simulink model "ADI"  (R2019b)
settings: Solver=FixedStepAuto  StartTime=0.0  StopTime=10.0  FixedStep=fixedStepSize  RelTol=1e-3
undefined symbols (not defined in the file): ADI_evChangesDuration, ADI_notAlways1Horizon, ADI_outputTorqueBound, ADI_subsystem1_downThreshold1, ADI_subsystem1_downThreshold2, ADI_subsystem1_downThreshold3, ADI_subsystem1_downThreshold4, ADI_subsystem1_evChangesDuration, ADI_subsystem1_gearOption1, ADI_subsystem1_gearOption2, ADI_subsystem1_speedThreshold, ADI_subsystem2_evChangesDuration, ADI_subsystem2_gear1, ADI_subsystem2_gear2, ADI_subsystem2_notAlwaysHorizon, ADI_subsystem2_speedMin, ADI_subsystem3_downThreshold, ADI_subsystem3_gear, ADI_subsystem3_gearSelectionState, ADI_subsystem3_impellerTorque, ADI_subsystem3_RPM, ADI_subsystem3_upThreshold, ADI_subsystem4_downThreshold, ADI_subsystem4_gear, ADI_subsystem4_gearSelectionState, ADI_subsystem4_notAlways1Horizon, ADI_subsystem4_notAlwaysHorizon, ADI_subsystem4_RPM, ADI_subsystem4_throttle, ADI_subsystem4_upThreshold, ADI_subsystem5_evChanges1Duration, ADI_subsystem5_evChangesDuration, ADI_subsystem5_notAlwaysHorizon, ADI_subsystem5_speedThreshold, fixedStepSize
libraries: simulink x11
settings Model: Creator=JEDDELAN  LastModifiedBy=alex
settings DataIOCC: ReturnWorkspaceOutputs=off
settings DebuggingCC: ArithmeticOperatorsInVariantConditions=warning
settings SFSimCC: SimUseLocalCustomCode=off  CustomCodeUndefinedFunction=UseInterfaceOnly
settings RTWCC: RTWUseLocalCustomCode=off

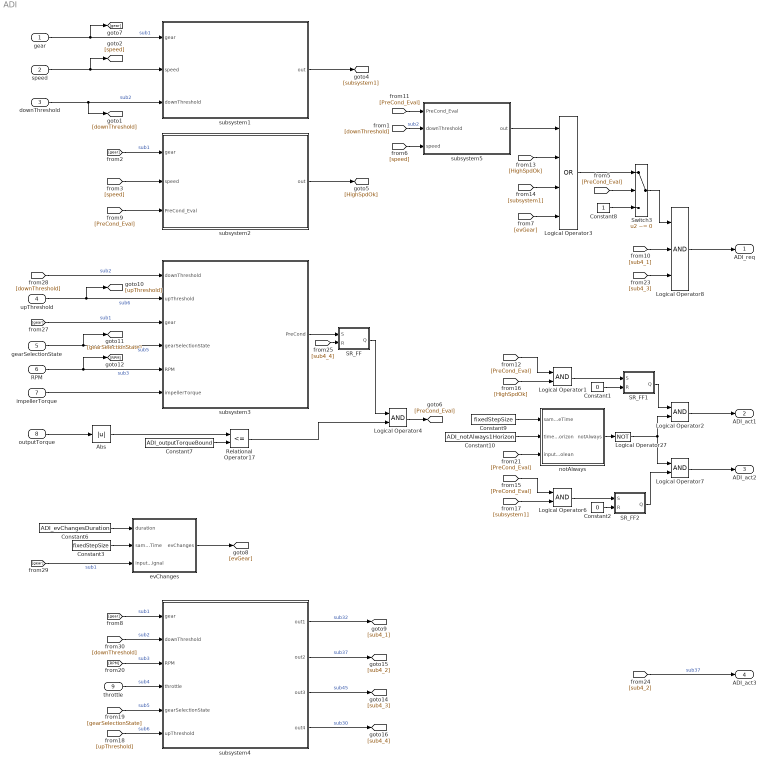
== system ADI ==
  gear : Inport
  speed : Inport  Port=2
  downThreshold : Inport  Port=3
  upThreshold : Inport  Port=4
  gearSelectionState : Inport  Port=5
  RPM : Inport  Port=6
  impellerTorque : Inport  Port=7
  outputTorque : Inport  Port=8
  throttle : Inport  Port=9
  Abs : Abs
  Constant1 : Constant  Value=0  OutDataTypeStr=boolean
  Constant10 : Constant  Value=ADI_notAlways1Horizon
  Constant2 : Constant  Value=0  OutDataTypeStr=boolean
  Constant3 : Constant  Value=fixedStepSize
  Constant6 : Constant  Value=ADI_evChangesDuration
  Constant7 : Constant  Value=ADI_outputTorqueBound
  Constant8 : Constant
  Constant9 : Constant  Value=fixedStepSize
  Logical Operator{1..2,4,6..7} (5 alike) : Logic  AllPortsSameDT=off  OutDataTypeStr=boolean
  Logical Operator27 : Logic  Operator=NOT  AllPortsSameDT=off  OutDataTypeStr=boolean
  Logical Operator3 : Logic  Operator=OR  Inputs=4  AllPortsSameDT=off  OutDataTypeStr=boolean
  Logical Operator8 : Logic  Inputs=3  AllPortsSameDT=off  OutDataTypeStr=boolean
  Relational Operator17 : RelationalOperator  Operator=<=  OutDataTypeStr=boolean  RndMeth=Nearest
  SR_FF : Subsystem
      settings: CopyFcn=set_param(gcbh,'LinkStatus','none');
  SR_FF1 : Subsystem
      settings: CopyFcn=set_param(gcbh,'LinkStatus','none');
  SR_FF2 : Subsystem
      settings: CopyFcn=set_param(gcbh,'LinkStatus','none');
  Switch3 : Switch  Criteria=u2 ~= 0
  evChanges : Subsystem
      settings: CopyFcn=set_param(gcbh,'LinkStatus','none');
  notAlways : Subsystem
      settings: CopyFcn=set_param(gcbh,'LinkStatus','none');
  subsystem1 : Subsystem
  subsystem2 : Subsystem
  subsystem3 : Subsystem
  subsystem4 : Subsystem
  subsystem5 : Subsystem
  ADI_req : Outport  OutDataTypeStr=boolean  PortDimensions=1  VectorParamsAs1DForOutWhenUnconnected=off
  ADI_act1 : Outport  Port=2  OutDataTypeStr=boolean  PortDimensions=1  VectorParamsAs1DForOutWhenUnconnected=off
  ADI_act2 : Outport  Port=3  OutDataTypeStr=boolean  PortDimensions=1  VectorParamsAs1DForOutWhenUnconnected=off
  ADI_act3 : Outport  Port=4  OutDataTypeStr=boolean  PortDimensions=1  VectorParamsAs1DForOutWhenUnconnected=off
  wires:
  evChanges/1(evChanges) -> [evGear]
  [gear] -> evChanges/3(inputSignal)  "sub1"
  Relational Operator17/1 -> Logical Operator4/2
  subsystem4/2(out2) -> [sub4_2]  "sub37"
  Constant10/1 -> notAlways/2(timeHorizon)
  [downThreshold] -> subsystem3/1(downThreshold)  "sub2"
  SR_FF/1(Q) -> Logical Operator4/1
  subsystem4/4(out4) -> [sub4_4]  "sub30"
  [subsystem1] -> Logical Operator6/2
  subsystem3/1(PreCond) -> SR_FF/1(S)
  [sub4_4] -> SR_FF/2(R)
  [downThreshold] -> subsystem5/2(downThreshold)  "sub2"
  [HighSpdOk] -> Logical Operator1/2
  [upThreshold] -> subsystem4/6(upThreshold)  "sub6"
  Logical Operator3/1 -> Switch3/1
  subsystem4/3(out3) -> [sub4_3]  "sub45"
  impellerTorque/1 -> subsystem3/6(impellerTorque)
  [sub4_3] -> Logical Operator8/3
  [PreCond_Eval] -> subsystem2/3(PreCond_Eval)
  [sub4_1] -> Logical Operator8/2
  [gear] -> subsystem4/1(gear)  "sub1"
  Abs/1 -> Relational Operator17/1
  [downThreshold] -> subsystem4/2(downThreshold)  "sub2"
  Constant6/1 -> evChanges/1(duration)
  [gear] -> subsystem2/1(gear)  "sub1"
  Logical Operator27/1 -> Logical Operator2/2, Logical Operator7/1
  speed/1 -> subsystem1/2("speed "), [speed]
  [speed] -> subsystem2/2(speed)
  gear/1 -> subsystem1/1(gear), [gear]  "sub1"
  [gear] -> subsystem3/3(gear)  "sub1"
  [sub4_2] -> ADI_act3/1  "sub37"
  [RPM] -> subsystem4/3(RPM)  "sub3"
  notAlways/1(notAlways) -> Logical Operator27/1
  [speed] -> subsystem5/3(speed)
  gearSelectionState/1 -> [gearSelectionState], subsystem3/4(gearSelectionState)  "sub5"
  Logical Operator8/1 -> ADI_req/1
  Logical Operator7/1 -> ADI_act2/1
  Logical Operator6/1 -> SR_FF2/1(S)
  RPM/1 -> [RPM], subsystem3/5(RPM)  "sub3"
  Constant7/1 -> Relational Operator17/2
  upThreshold/1 -> subsystem3/2(upThreshold), [upThreshold]  "sub6"
  downThreshold/1 -> subsystem1/3(downThreshold), [downThreshold]  "sub2"
  [PreCond_Eval] -> Switch3/2
  [gearSelectionState] -> subsystem4/5(gearSelectionState)  "sub5"
  throttle/1 -> subsystem4/4(throttle)  "sub4"
  Constant2/1 -> SR_FF2/2(R)
  [PreCond_Eval] -> Logical Operator1/1
  subsystem2/1(out) -> [HighSpdOk]
  Constant9/1 -> notAlways/1(sampleTime)
  Logical Operator4/1 -> [PreCond_Eval]
  subsystem1/1(out) -> [subsystem1]
  [PreCond_Eval] -> Logical Operator6/1
  [evGear] -> Logical Operator3/4
  SR_FF2/1(Q) -> Logical Operator7/2
  SR_FF1/1(Q) -> Logical Operator2/1
  Constant8/1 -> Switch3/3
  [HighSpdOk] -> Logical Operator3/2
  Logical Operator2/1 -> ADI_act1/1
  [subsystem1] -> Logical Operator3/3
  Switch3/1 -> Logical Operator8/1
  [PreCond_Eval] -> subsystem5/1(PreCond_Eval)
  subsystem4/1(out1) -> [sub4_1]  "sub32"
  Logical Operator1/1 -> SR_FF1/1(S)
  subsystem5/1(out) -> Logical Operator3/1
  [PreCond_Eval] -> notAlways/3(inputBoolean)
  outputTorque/1 -> Abs/1
  Constant3/1 -> evChanges/2(sampleTime)
  Constant1/1 -> SR_FF1/2(R)

== system ADI/SR_FF ==
  S : Inport  OutDataTypeStr=boolean
  R : Inport  Port=2  OutDataTypeStr=boolean
  LogOp1 : Logic  Tag=struct('inputs','1','comment',struct('text','','placement',1),'logdata',struct('maxnumvals',4096,'plotchannels',[],'loggingmode',3,'channels',1),'operator','NOT','output',struct('class','default','description','','address','','unit','-','name','$S_$B','variable','','type','Bool'),'date',733638.68643228011,'scalingvalid',0)  Operator=NOT  Inputs=1  OutDataTypeStr=boolean
  LogOp2 : Logic  Tag=struct('inputs','2','comment',struct('text','','placement',1),'logdata',struct('maxnumvals',4096,'plotchannels',[],'loggingmode',3,'channels',1),'operator','AND','output',struct('class','default','description','','address','','unit','-','name','$S_$B','variable','','type','Bool'),'date',733638.68643680552,'scalingvalid',0)  Operator=OR  OutDataTypeStr=boolean
  LogOp3 : Logic  Tag=struct('inputs','2','comment',struct('text','','placement',1),'logdata',struct('maxnumvals',4096,'plotchannels',[],'loggingmode',3,'channels',1),'operator','OR','output',struct('class','default','description','','address','','unit','-','name','$S_$B','variable','','type','Bool'),'date',733638.68644151615,'scalingvalid',0)  OutDataTypeStr=boolean
  UnitDelay1 : UnitDelay  Tag=struct('comment',struct('text','','placement',1),'logdata',struct('maxnumvals',4096,'plotchannels',[],'loggingmode',3,'channels',1),'output',struct('width',1,'name','$S_$B','unit','','type','Bool','offset',0,'max',NaN,'min',NaN,'freeze',1,'lsb',1,'arb',0,'class','default','address','','description','','autoscalingmode',1,'lowerheadroom',1,'upperheadroom',1,'headroomunit','bit','checkmin',0,'checkmax',0,'show',0,'variable','','scaling','','keepdatatype',1,'castoutput',0),'state',struct('variable','','description','','name','X_$S_$B','width',1,'address','','max',NaN,'min',NaN,'class','default','type','Bool','scaling','','lsb',1,'offset',0,'arb',0,'freeze',1,'unit','','initial','0'),'dt','-1','date',733638.68644640048,'scalingvalid',0)  SampleTime=-1  HasFrameUpgradeWarning=on
  Q : Outport  OutDataTypeStr=boolean  VectorParamsAs1DForOutWhenUnconnected=off
  wires:
  UnitDelay1/1 -> LogOp2/1  "UnitDelay1_3"
  S/1 -> LogOp2/2
  R/1 -> LogOp1/1
  LogOp2/1 -> LogOp3/1
  LogOp1/1 -> LogOp3/2
  LogOp3/1 -> UnitDelay1/1, Q/1

== system ADI/SR_FF1 ==
  S : Inport  OutDataTypeStr=boolean
  R : Inport  Port=2  OutDataTypeStr=boolean
  LogOp1 : Logic  Tag=struct('inputs','1','comment',struct('text','','placement',1),'logdata',struct('maxnumvals',4096,'plotchannels',[],'loggingmode',3,'channels',1),'operator','NOT','output',struct('class','default','description','','address','','unit','-','name','$S_$B','variable','','type','Bool'),'date',733638.68643228011,'scalingvalid',0)  Operator=NOT  Inputs=1  OutDataTypeStr=boolean
  LogOp2 : Logic  Tag=struct('inputs','2','comment',struct('text','','placement',1),'logdata',struct('maxnumvals',4096,'plotchannels',[],'loggingmode',3,'channels',1),'operator','AND','output',struct('class','default','description','','address','','unit','-','name','$S_$B','variable','','type','Bool'),'date',733638.68643680552,'scalingvalid',0)  Operator=OR  OutDataTypeStr=boolean
  LogOp3 : Logic  Tag=struct('inputs','2','comment',struct('text','','placement',1),'logdata',struct('maxnumvals',4096,'plotchannels',[],'loggingmode',3,'channels',1),'operator','OR','output',struct('class','default','description','','address','','unit','-','name','$S_$B','variable','','type','Bool'),'date',733638.68644151615,'scalingvalid',0)  OutDataTypeStr=boolean
  UnitDelay1 : UnitDelay  Tag=struct('comment',struct('text','','placement',1),'logdata',struct('maxnumvals',4096,'plotchannels',[],'loggingmode',3,'channels',1),'output',struct('width',1,'name','$S_$B','unit','','type','Bool','offset',0,'max',NaN,'min',NaN,'freeze',1,'lsb',1,'arb',0,'class','default','address','','description','','autoscalingmode',1,'lowerheadroom',1,'upperheadroom',1,'headroomunit','bit','checkmin',0,'checkmax',0,'show',0,'variable','','scaling','','keepdatatype',1,'castoutput',0),'state',struct('variable','','description','','name','X_$S_$B','width',1,'address','','max',NaN,'min',NaN,'class','default','type','Bool','scaling','','lsb',1,'offset',0,'arb',0,'freeze',1,'unit','','initial','0'),'dt','-1','date',733638.68644640048,'scalingvalid',0)  SampleTime=-1  HasFrameUpgradeWarning=on
  Q : Outport  OutDataTypeStr=boolean  VectorParamsAs1DForOutWhenUnconnected=off
  wires:
  UnitDelay1/1 -> LogOp2/1
  S/1 -> LogOp2/2
  R/1 -> LogOp1/1
  LogOp2/1 -> LogOp3/1
  LogOp1/1 -> LogOp3/2
  LogOp3/1 -> UnitDelay1/1, Q/1

== system ADI/SR_FF2 ==
  S : Inport  OutDataTypeStr=boolean
  R : Inport  Port=2  OutDataTypeStr=boolean
  LogOp1 : Logic  Tag=struct('inputs','1','comment',struct('text','','placement',1),'logdata',struct('maxnumvals',4096,'plotchannels',[],'loggingmode',3,'channels',1),'operator','NOT','output',struct('class','default','description','','address','','unit','-','name','$S_$B','variable','','type','Bool'),'date',733638.68643228011,'scalingvalid',0)  Operator=NOT  Inputs=1  OutDataTypeStr=boolean
  LogOp2 : Logic  Tag=struct('inputs','2','comment',struct('text','','placement',1),'logdata',struct('maxnumvals',4096,'plotchannels',[],'loggingmode',3,'channels',1),'operator','AND','output',struct('class','default','description','','address','','unit','-','name','$S_$B','variable','','type','Bool'),'date',733638.68643680552,'scalingvalid',0)  Operator=OR  OutDataTypeStr=boolean
  LogOp3 : Logic  Tag=struct('inputs','2','comment',struct('text','','placement',1),'logdata',struct('maxnumvals',4096,'plotchannels',[],'loggingmode',3,'channels',1),'operator','OR','output',struct('class','default','description','','address','','unit','-','name','$S_$B','variable','','type','Bool'),'date',733638.68644151615,'scalingvalid',0)  OutDataTypeStr=boolean
  UnitDelay1 : UnitDelay  Tag=struct('comment',struct('text','','placement',1),'logdata',struct('maxnumvals',4096,'plotchannels',[],'loggingmode',3,'channels',1),'output',struct('width',1,'name','$S_$B','unit','','type','Bool','offset',0,'max',NaN,'min',NaN,'freeze',1,'lsb',1,'arb',0,'class','default','address','','description','','autoscalingmode',1,'lowerheadroom',1,'upperheadroom',1,'headroomunit','bit','checkmin',0,'checkmax',0,'show',0,'variable','','scaling','','keepdatatype',1,'castoutput',0),'state',struct('variable','','description','','name','X_$S_$B','width',1,'address','','max',NaN,'min',NaN,'class','default','type','Bool','scaling','','lsb',1,'offset',0,'arb',0,'freeze',1,'unit','','initial','0'),'dt','-1','date',733638.68644640048,'scalingvalid',0)  SampleTime=-1  HasFrameUpgradeWarning=on
  Q : Outport  OutDataTypeStr=boolean  VectorParamsAs1DForOutWhenUnconnected=off
  wires:
  UnitDelay1/1 -> LogOp2/1
  S/1 -> LogOp2/2
  R/1 -> LogOp1/1
  LogOp2/1 -> LogOp3/1
  LogOp1/1 -> LogOp3/2
  LogOp3/1 -> UnitDelay1/1, Q/1

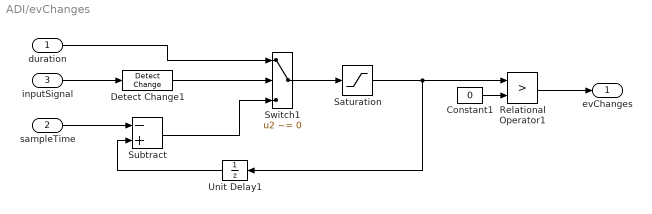
== system ADI/evChanges ==
  duration : Inport
  sampleTime : Inport  Port=2
  inputSignal : Inport  Port=3
  Constant1 : Constant  Value=0
  Detect Change1 : simulink/Logic and Bit Operations/Detect Change  vinit=0  OutDataTypeStr=boolean
  Relational Operator1 : RelationalOperator  Operator=>  OutDataTypeStr=boolean  RndMeth=Nearest
  Saturation : Saturate  UpperLimit=Inf  LowerLimit=0
  Subtract : Sum  Inputs=-+
  Switch1 : Switch  Criteria=u2 ~= 0
  Unit Delay1 : UnitDelay  SampleTime=-1  HasFrameUpgradeWarning=on
  evChanges : Outport  VectorParamsAs1DForOutWhenUnconnected=off
  wires:
  Detect Change1/1 -> Switch1/2
  duration/1 -> Switch1/1
  Switch1/1 -> Saturation/1
  inputSignal/1 -> Detect Change1/1
  Constant1/1 -> Relational Operator1/2
  Subtract/1 -> Switch1/3
  Saturation/1 -> Relational Operator1/1, Unit Delay1/1
  Unit Delay1/1 -> Subtract/2
  Relational Operator1/1 -> evChanges/1
  sampleTime/1 -> Subtract/1

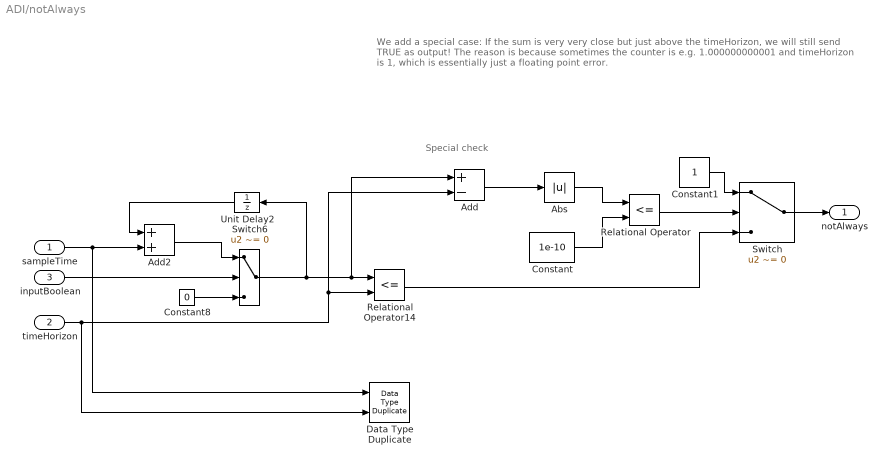
== system ADI/notAlways ==
  note: Special check
  note: We add a special case:
      | If the sum is very very close but just above the timeHorizon, we will still send TRUE as output!
      |
      | The reason is because sometimes the counter is e.g. 1.000000000001 and timeHorizon is 1, which is essentially just a floating point error.
  sampleTime : Inport
  timeHorizon : Inport  Port=2
  inputBoolean : Inport  Port=3
  Abs : Abs
  Add : Sum  Inputs=+-
  Add2 : Sum
  Constant : Constant  Value=1e-10
  Constant1 : Constant  OutDataTypeStr=boolean
  Constant8 : Constant  Value=0  OutDataTypeStr=Inherit: Inherit via back propagation
  Data Type Duplicate : DataTypeDuplicate
  Relational Operator : RelationalOperator  Operator=<=  OutDataTypeStr=boolean  RndMeth=Simplest
  Relational Operator14 : RelationalOperator  Operator=<=  OutDataTypeStr=boolean  RndMeth=Nearest
  Switch : Switch  Criteria=u2 ~= 0
  Switch6 : Switch  Criteria=u2 ~= 0
  Unit Delay2 : UnitDelay  SampleTime=-1  HasFrameUpgradeWarning=on
  notAlways : Outport  VectorParamsAs1DForOutWhenUnconnected=off
  wires:
  Switch6/1 -> Add/1, Relational Operator14/1, Unit Delay2/1
  timeHorizon/1 -> Add/2, Relational Operator14/2, Data Type Duplicate/2
  Relational Operator14/1 -> Switch/3
  Unit Delay2/1 -> Add2/1
  Add2/1 -> Switch6/1
  sampleTime/1 -> Add2/2, Data Type Duplicate/1
  Constant8/1 -> Switch6/3
  inputBoolean/1 -> Switch6/2
  Add/1 -> Abs/1
  Abs/1 -> Relational Operator/1
  Constant/1 -> Relational Operator/2
  Relational Operator/1 -> Switch/2
  Constant1/1 -> Switch/1
  Switch/1 -> notAlways/1

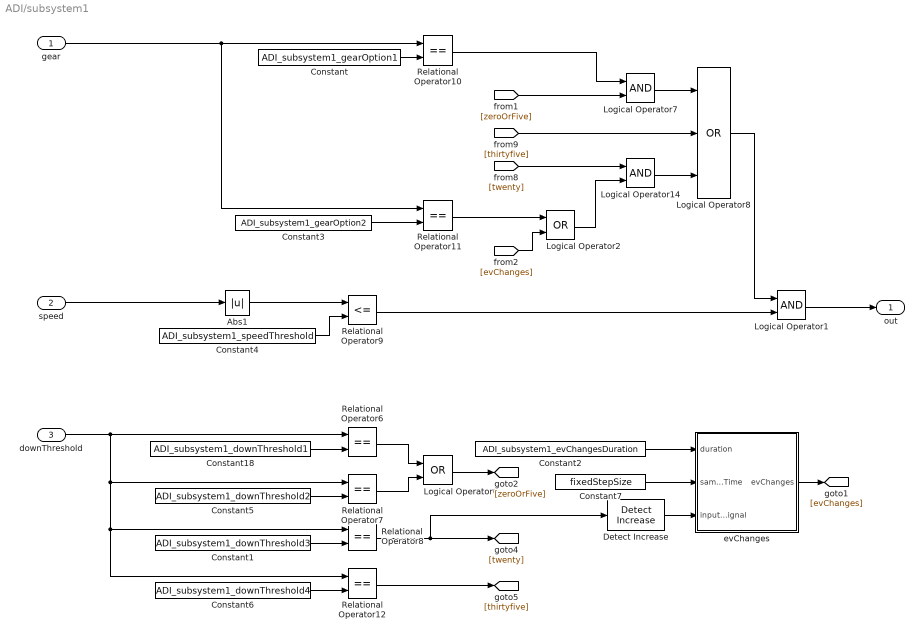
== system ADI/subsystem1 ==
  gear : Inport  Interpolate=off
  "speed " : Inport  Port=2
  downThreshold : Inport  Port=3
  Abs1 : Abs
  Constant : Constant  Value=ADI_subsystem1_gearOption1
  Constant1 : Constant  Value=ADI_subsystem1_downThreshold3
  Constant18 : Constant  Value=ADI_subsystem1_downThreshold1
  Constant2 : Constant  Value=ADI_subsystem1_evChangesDuration
  Constant3 : Constant  Value=ADI_subsystem1_gearOption2
  Constant4 : Constant  Value=ADI_subsystem1_speedThreshold
  Constant5 : Constant  Value=ADI_subsystem1_downThreshold2
  Constant6 : Constant  Value=ADI_subsystem1_downThreshold4
  Constant7 : Constant  Value=fixedStepSize
  Detect Increase : simulink/Logic and Bit Operations/Detect Increase  vinit=0.0  OutDataTypeStr=boolean
  Logical Operator1 : Logic  AllPortsSameDT=off  OutDataTypeStr=boolean
  Logical Operator14 : Logic  AllPortsSameDT=off  OutDataTypeStr=boolean
  Logical Operator2 : Logic  Operator=OR  AllPortsSameDT=off  OutDataTypeStr=boolean
  Logical Operator6 : Logic  Operator=OR  AllPortsSameDT=off  OutDataTypeStr=boolean
  Logical Operator7 : Logic  AllPortsSameDT=off  OutDataTypeStr=boolean
  Logical Operator8 : Logic  Operator=OR  Inputs=3  AllPortsSameDT=off  OutDataTypeStr=boolean
  Relational Operator{6..8,10..12} (6 alike) : RelationalOperator  Operator===  OutDataTypeStr=boolean  RndMeth=Nearest
  Relational Operator9 : RelationalOperator  Operator=<=  OutDataTypeStr=boolean  RndMeth=Nearest
  evChanges : Subsystem
      settings: CopyFcn=set_param(gcbh,'LinkStatus','none');
  out : Outport  VectorParamsAs1DForOutWhenUnconnected=off
  wires:
  Detect Increase/1 -> evChanges/3(inputSignal)
  Constant7/1 -> evChanges/2(sampleTime)
  evChanges/1(evChanges) -> [evChanges]
  [evChanges] -> Logical Operator2/2
  Logical Operator2/1 -> Logical Operator14/2
  Logical Operator1/1 -> out/1
  "speed "/1 -> Abs1/1
  Relational Operator9/1 -> Logical Operator1/2
  Abs1/1 -> Relational Operator9/1
  [twenty] -> Logical Operator14/1
  Logical Operator8/1 -> Logical Operator1/1
  [thirtyfive] -> Logical Operator8/2
  Logical Operator7/1 -> Logical Operator8/1
  Relational Operator11/1 -> Logical Operator2/1
  Relational Operator10/1 -> Logical Operator7/1
  [zeroOrFive] -> Logical Operator7/2
  Relational Operator12/1 -> [thirtyfive]
  Constant6/1 -> Relational Operator12/2
  gear/1 -> Relational Operator11/1, Relational Operator10/1
  Constant3/1 -> Relational Operator11/2
  Constant/1 -> Relational Operator10/2
  Logical Operator14/1 -> Logical Operator8/3
  Constant4/1 -> Relational Operator9/2
  Constant1/1 -> Relational Operator8/2
  Relational Operator8/1 -> Detect Increase/1, [twenty]
  Logical Operator6/1 -> [zeroOrFive]
  Relational Operator6/1 -> Logical Operator6/1
  Relational Operator7/1 -> Logical Operator6/2
  Constant5/1 -> Relational Operator7/2
  Constant18/1 -> Relational Operator6/2
  downThreshold/1 -> Relational Operator6/1, Relational Operator7/1, Relational Operator8/1, Relational Operator12/1
  Constant2/1 -> evChanges/1(duration)

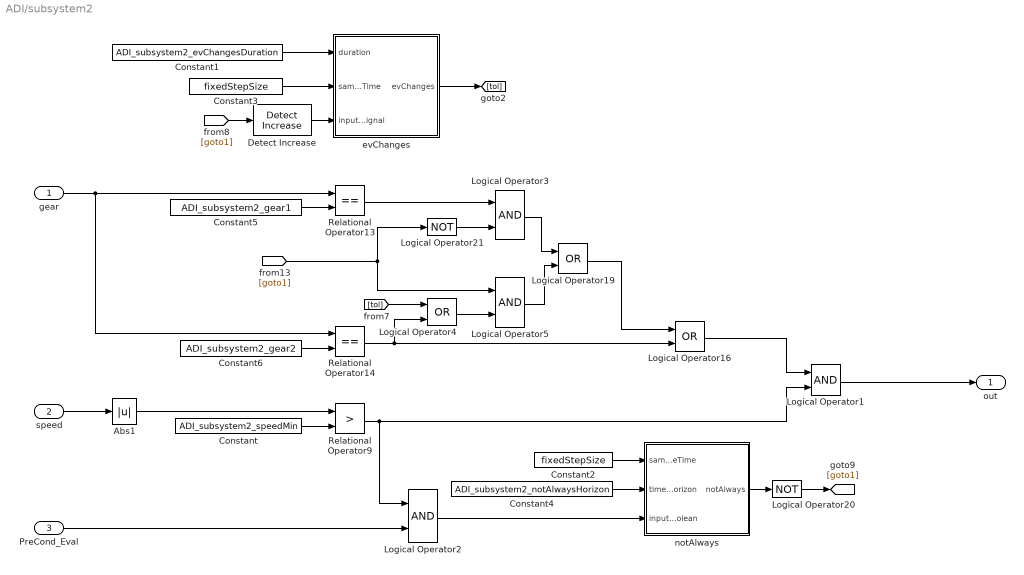
== system ADI/subsystem2 ==
  gear : Inport
  speed : Inport  Port=2
  PreCond_Eval : Inport  Port=3
  Abs1 : Abs
  Constant : Constant  Value=ADI_subsystem2_speedMin
  Constant1 : Constant  Value=ADI_subsystem2_evChangesDuration
  Constant2 : Constant  Value=fixedStepSize
  Constant3 : Constant  Value=fixedStepSize
  Constant4 : Constant  Value=ADI_subsystem2_notAlwaysHorizon
  Constant5 : Constant  Value=ADI_subsystem2_gear1
  Constant6 : Constant  Value=ADI_subsystem2_gear2
  Detect Increase : simulink/Logic and Bit Operations/Detect Increase  vinit=0.0  OutDataTypeStr=boolean
  Logical Operator{1..3,5} (4 alike) : Logic  AllPortsSameDT=off  OutDataTypeStr=boolean
  Logical Operator16 : Logic  Operator=OR  AllPortsSameDT=off  OutDataTypeStr=boolean
  Logical Operator19 : Logic  Operator=OR  AllPortsSameDT=off  OutDataTypeStr=boolean
  Logical Operator20 : Logic  Operator=NOT  AllPortsSameDT=off  OutDataTypeStr=boolean
  Logical Operator21 : Logic  Operator=NOT  AllPortsSameDT=off  OutDataTypeStr=boolean
  Logical Operator4 : Logic  Operator=OR  AllPortsSameDT=off  OutDataTypeStr=boolean
  Relational Operator13 : RelationalOperator  Operator===  OutDataTypeStr=boolean  RndMeth=Nearest
  Relational Operator14 : RelationalOperator  Operator===  OutDataTypeStr=boolean  RndMeth=Nearest
  Relational Operator9 : RelationalOperator  Operator=>  OutDataTypeStr=boolean  RndMeth=Nearest
  evChanges : Subsystem
      settings: CopyFcn=set_param(gcbh,'LinkStatus','none');
  notAlways : Subsystem
      settings: CopyFcn=set_param(gcbh,'LinkStatus','none');
  out : Outport  VectorParamsAs1DForOutWhenUnconnected=off
  wires:
  Detect Increase/1 -> evChanges/3(inputSignal)
  Logical Operator20/1 -> [goto1]
  Logical Operator2/1 -> notAlways/3(inputBoolean)
  Logical Operator4/1 -> Logical Operator5/2
  [goto1] -> Detect Increase/1
  Constant3/1 -> evChanges/2(sampleTime)
  Constant1/1 -> evChanges/1(duration)
  evChanges/1(evChanges) -> [tol]
  [tol] -> Logical Operator4/1
  Logical Operator1/1 -> out/1
  PreCond_Eval/1 -> Logical Operator2/2
  Relational Operator9/1 -> Logical Operator1/2, Logical Operator2/1
  Constant/1 -> Relational Operator9/2
  Abs1/1 -> Relational Operator9/1
  speed/1 -> Abs1/1
  Logical Operator16/1 -> Logical Operator1/1
  Logical Operator21/1 -> Logical Operator3/2
  [goto1] -> Logical Operator5/1, Logical Operator21/1
  Constant5/1 -> Relational Operator13/2
  notAlways/1(notAlways) -> Logical Operator20/1
  Constant4/1 -> notAlways/2(timeHorizon)
  Constant2/1 -> notAlways/1(sampleTime)
  Relational Operator13/1 -> Logical Operator3/1
  Logical Operator3/1 -> Logical Operator19/1
  Logical Operator5/1 -> Logical Operator19/2
  Logical Operator19/1 -> Logical Operator16/1
  Relational Operator14/1 -> Logical Operator4/2, Logical Operator16/2
  Constant6/1 -> Relational Operator14/2
  gear/1 -> Relational Operator13/1, Relational Operator14/1

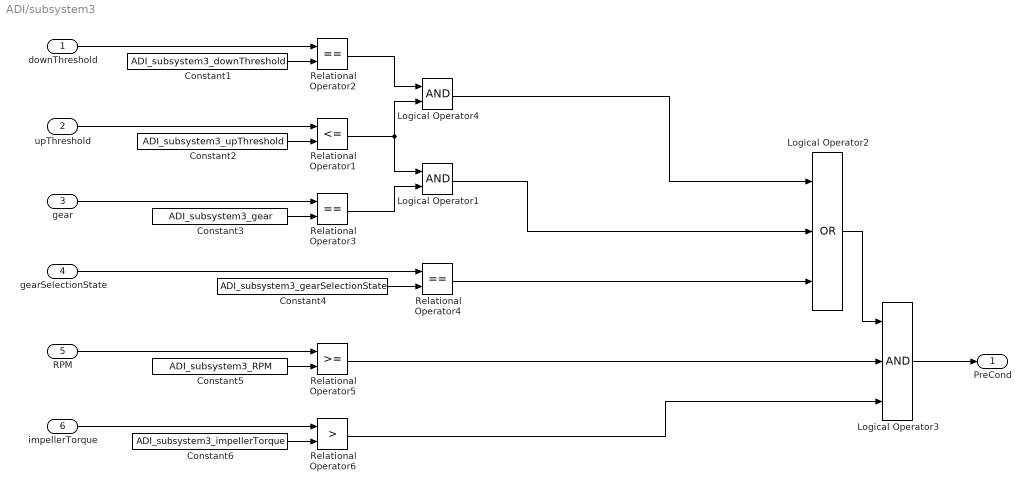
== system ADI/subsystem3 ==
  downThreshold : Inport
  upThreshold : Inport  Port=2
  gear : Inport  Port=3
  gearSelectionState : Inport  Port=4
  RPM : Inport  Port=5
  impellerTorque : Inport  Port=6
  Constant1 : Constant  Value=ADI_subsystem3_downThreshold
  Constant2 : Constant  Value=ADI_subsystem3_upThreshold
  Constant3 : Constant  Value=ADI_subsystem3_gear
  Constant4 : Constant  Value=ADI_subsystem3_gearSelectionState
  Constant5 : Constant  Value=ADI_subsystem3_RPM
  Constant6 : Constant  Value=ADI_subsystem3_impellerTorque
  Logical Operator1 : Logic  AllPortsSameDT=off  OutDataTypeStr=boolean
  Logical Operator2 : Logic  Operator=OR  Inputs=3  AllPortsSameDT=off  OutDataTypeStr=boolean
  Logical Operator3 : Logic  Inputs=3  AllPortsSameDT=off  OutDataTypeStr=boolean
  Logical Operator4 : Logic  AllPortsSameDT=off  OutDataTypeStr=boolean
  Relational Operator1 : RelationalOperator  Operator=<=  OutDataTypeStr=boolean  RndMeth=Nearest
  Relational Operator2 : RelationalOperator  Operator===  OutDataTypeStr=boolean  RndMeth=Nearest
  Relational Operator3 : RelationalOperator  Operator===  OutDataTypeStr=boolean  RndMeth=Nearest
  Relational Operator4 : RelationalOperator  Operator===  OutDataTypeStr=boolean  RndMeth=Nearest
  Relational Operator5 : RelationalOperator  OutDataTypeStr=boolean  RndMeth=Nearest
  Relational Operator6 : RelationalOperator  Operator=>  OutDataTypeStr=boolean  RndMeth=Nearest
  PreCond : Outport  VectorParamsAs1DForOutWhenUnconnected=off
  wires:
  Logical Operator2/1 -> Logical Operator3/1
  Logical Operator3/1 -> PreCond/1
  Relational Operator5/1 -> Logical Operator3/2
  Constant5/1 -> Relational Operator5/2
  RPM/1 -> Relational Operator5/1
  Relational Operator4/1 -> Logical Operator2/3
  Constant4/1 -> Relational Operator4/2
  gearSelectionState/1 -> Relational Operator4/1
  Relational Operator3/1 -> Logical Operator1/2
  Relational Operator1/1 -> Logical Operator1/1, Logical Operator4/2
  Relational Operator2/1 -> Logical Operator4/1
  Logical Operator4/1 -> Logical Operator2/1
  Logical Operator1/1 -> Logical Operator2/2
  Constant3/1 -> Relational Operator3/2
  gear/1 -> Relational Operator3/1
  Constant2/1 -> Relational Operator1/2
  upThreshold/1 -> Relational Operator1/1
  downThreshold/1 -> Relational Operator2/1
  Constant1/1 -> Relational Operator2/2
  Constant6/1 -> Relational Operator6/2
  impellerTorque/1 -> Relational Operator6/1
  Relational Operator6/1 -> Logical Operator3/3

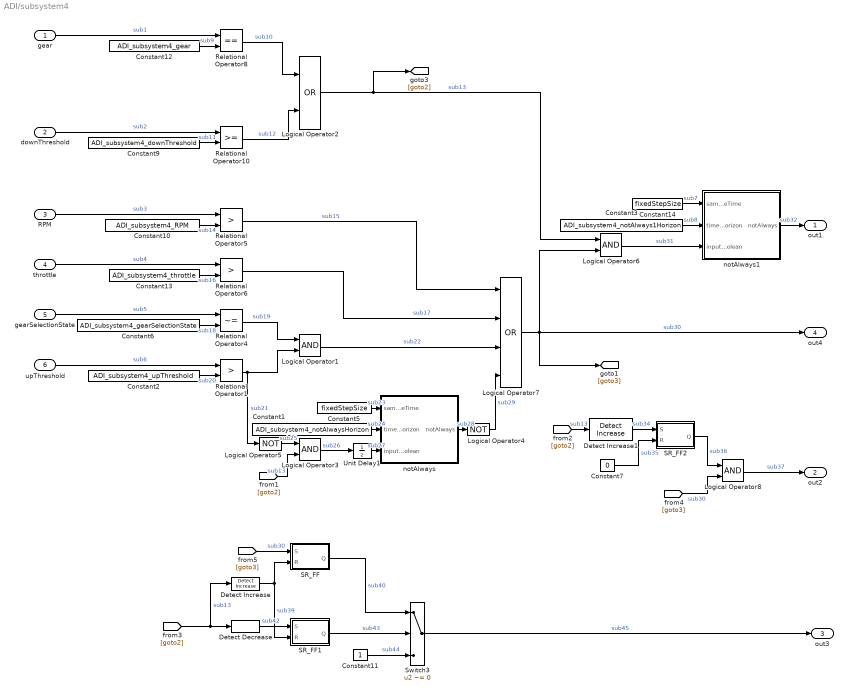
== system ADI/subsystem4 ==
  gear : Inport  Interpolate=off
  downThreshold : Inport  Port=2
  RPM : Inport  Port=3
  throttle : Inport  Port=4
  gearSelectionState : Inport  Port=5
  upThreshold : Inport  Port=6
  Constant1 : Constant  Value=ADI_subsystem4_notAlwaysHorizon
  Constant10 : Constant  Value=ADI_subsystem4_RPM
  Constant11 : Constant
  Constant12 : Constant  Value=ADI_subsystem4_gear
  Constant13 : Constant  Value=ADI_subsystem4_throttle
  Constant14 : Constant  Value=fixedStepSize
  Constant2 : Constant  Value=ADI_subsystem4_upThreshold
  Constant3 : Constant  Value=ADI_subsystem4_notAlways1Horizon
  Constant5 : Constant  Value=fixedStepSize
  Constant6 : Constant  Value=ADI_subsystem4_gearSelectionState
  Constant7 : Constant  Value=0  OutDataTypeStr=boolean
  Constant9 : Constant  Value=ADI_subsystem4_downThreshold
  Detect Decrease : simulink/Logic and Bit Operations/Detect Decrease  vinit=0.0  OutDataTypeStr=boolean
  Detect Increase : simulink/Logic and Bit Operations/Detect Increase  vinit=0.0  OutDataTypeStr=boolean
  Detect Increase1 : simulink/Logic and Bit Operations/Detect Increase  vinit=0.0  OutDataTypeStr=boolean
  Logical Operator{1,3,6,8} (4 alike) : Logic  AllPortsSameDT=off  OutDataTypeStr=boolean
  Logical Operator2 : Logic  Operator=OR  AllPortsSameDT=off  OutDataTypeStr=boolean
  Logical Operator4 : Logic  Operator=NOT  AllPortsSameDT=off  OutDataTypeStr=boolean
  Logical Operator5 : Logic  Operator=NOT  AllPortsSameDT=off  OutDataTypeStr=boolean
  Logical Operator7 : Logic  Operator=OR  Inputs=4  AllPortsSameDT=off  OutDataTypeStr=boolean
  Relational Operator1 : RelationalOperator  Operator=>  OutDataTypeStr=boolean  RndMeth=Nearest
  Relational Operator10 : RelationalOperator  OutDataTypeStr=boolean  RndMeth=Nearest
  Relational Operator4 : RelationalOperator  Operator=~=  OutDataTypeStr=boolean  RndMeth=Nearest
  Relational Operator5 : RelationalOperator  Operator=>  OutDataTypeStr=boolean  RndMeth=Nearest
  Relational Operator6 : RelationalOperator  Operator=>  OutDataTypeStr=boolean  RndMeth=Nearest
  Relational Operator8 : RelationalOperator  Operator===  OutDataTypeStr=boolean  RndMeth=Nearest
  SR_FF : Subsystem
      settings: CopyFcn=set_param(gcbh,'LinkStatus','none');
  SR_FF1 : Subsystem
      settings: CopyFcn=set_param(gcbh,'LinkStatus','none');
  SR_FF2 : Subsystem
      settings: CopyFcn=set_param(gcbh,'LinkStatus','none');
  Switch3 : Switch  Criteria=u2 ~= 0
  Unit Delay1 : UnitDelay  SampleTime=-1  HasFrameUpgradeWarning=on
  notAlways : Subsystem
      settings: CopyFcn=set_param(gcbh,'LinkStatus','none');
  notAlways1 : Subsystem
      settings: CopyFcn=set_param(gcbh,'LinkStatus','none');
  out1 : Outport  VectorParamsAs1DForOutWhenUnconnected=off
  out2 : Outport  Port=2  VectorParamsAs1DForOutWhenUnconnected=off
  out3 : Outport  Port=3  VectorParamsAs1DForOutWhenUnconnected=off
  out4 : Outport  Port=4  VectorParamsAs1DForOutWhenUnconnected=off
  wires:
  Relational Operator6/1 -> Logical Operator7/2  "sub17"
  throttle/1 -> Relational Operator6/1  "sub4"
  Constant13/1 -> Relational Operator6/2  "sub16"
  upThreshold/1 -> Relational Operator1/1  "sub6"
  Constant2/1 -> Relational Operator1/2  "sub20"
  Logical Operator1/1 -> Logical Operator7/3  "sub22"
  Relational Operator1/1 -> Logical Operator1/2, Logical Operator5/1  "sub21"
  gearSelectionState/1 -> Relational Operator4/1  "sub5"
  Constant6/1 -> Relational Operator4/2  "sub18"
  Relational Operator4/1 -> Logical Operator1/1  "sub19"
  RPM/1 -> Relational Operator5/1  "sub3"
  Constant10/1 -> Relational Operator5/2  "sub14"
  Relational Operator5/1 -> Logical Operator7/1  "sub15"
  Constant5/1 -> notAlways/1(sampleTime)  "sub23"
  Constant1/1 -> notAlways/2(timeHorizon)  "sub24"
  gear/1 -> Relational Operator8/1  "sub1"
  Constant12/1 -> Relational Operator8/2  "sub9"
  Relational Operator8/1 -> Logical Operator2/1  "sub10"
  Logical Operator2/1 -> Logical Operator6/1, [goto2]  "sub13"
  downThreshold/1 -> Relational Operator10/1  "sub2"
  Constant9/1 -> Relational Operator10/2  "sub11"
  Relational Operator10/1 -> Logical Operator2/2  "sub12"
  Logical Operator3/1 -> Unit Delay1/1  "sub26"
  Logical Operator5/1 -> Logical Operator3/1  "sub25"
  Logical Operator7/1 -> out4/1, [goto3], Logical Operator6/2  "sub30"
  Logical Operator6/1 -> notAlways1/3(inputBoolean)  "sub31"
  notAlways1/1(notAlways) -> out1/1  "sub32"
  Constant14/1 -> notAlways1/1(sampleTime)  "sub7"
  Constant3/1 -> notAlways1/2(timeHorizon)  "sub8"
  Logical Operator4/1 -> Logical Operator7/4  "sub29"
  Constant7/1 -> SR_FF2/2(R)  "sub35"
  [goto2] -> Detect Increase1/1  "sub13"
  SR_FF2/1(Q) -> Logical Operator8/1  "sub36"
  Detect Increase1/1 -> SR_FF2/1(S)  "sub34"
  Logical Operator8/1 -> out2/1  "sub37"
  [goto2] -> Detect Increase/1, Detect Decrease/1  "sub13"
  [goto3] -> Logical Operator8/2  "sub30"
  Detect Decrease/1 -> SR_FF1/1(S)  "sub42"
  [goto3] -> SR_FF/1(S)  "sub30"
  Detect Increase/1 -> SR_FF1/2(R), SR_FF/2(R)  "sub39"
  SR_FF1/1(Q) -> Switch3/2  "sub43"
  SR_FF/1(Q) -> Switch3/1  "sub40"
  Constant11/1 -> Switch3/3  "sub44"
  Switch3/1 -> out3/1  "sub45"
  [goto2] -> Logical Operator3/2  "sub13"
  Unit Delay1/1 -> notAlways/3(inputBoolean)  "sub27"
  notAlways/1(notAlways) -> Logical Operator4/1  "sub28"

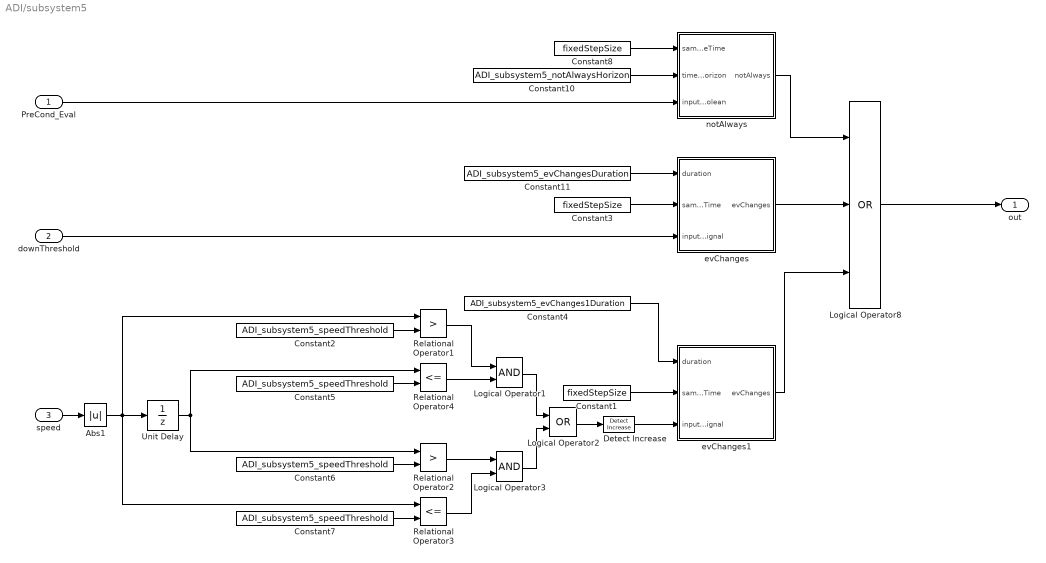
== system ADI/subsystem5 ==
  PreCond_Eval : Inport
  downThreshold : Inport  Port=2
  speed : Inport  Port=3
  Abs1 : Abs
  Constant1 : Constant  Value=fixedStepSize
  Constant10 : Constant  Value=ADI_subsystem5_notAlwaysHorizon
  Constant11 : Constant  Value=ADI_subsystem5_evChangesDuration
  Constant{2,5..7} (4 alike) : Constant  Value=ADI_subsystem5_speedThreshold
  Constant3 : Constant  Value=fixedStepSize
  Constant4 : Constant  Value=ADI_subsystem5_evChanges1Duration
  Constant8 : Constant  Value=fixedStepSize
  Detect Increase : simulink/Logic and Bit Operations/Detect Increase  vinit=0.0  OutDataTypeStr=boolean
  Logical Operator1 : Logic  AllPortsSameDT=off  OutDataTypeStr=boolean
  Logical Operator2 : Logic  Operator=OR  AllPortsSameDT=off  OutDataTypeStr=boolean
  Logical Operator3 : Logic  AllPortsSameDT=off  OutDataTypeStr=boolean
  Logical Operator8 : Logic  Operator=OR  Inputs=3  AllPortsSameDT=off  OutDataTypeStr=boolean
  Relational Operator1 : RelationalOperator  Operator=>  OutDataTypeStr=boolean  RndMeth=Nearest
  Relational Operator2 : RelationalOperator  Operator=>  OutDataTypeStr=boolean  RndMeth=Nearest
  Relational Operator3 : RelationalOperator  Operator=<=  OutDataTypeStr=boolean  RndMeth=Nearest
  Relational Operator4 : RelationalOperator  Operator=<=  OutDataTypeStr=boolean  RndMeth=Nearest
  Unit Delay : UnitDelay  SampleTime=-1  HasFrameUpgradeWarning=on
  evChanges : Subsystem
      settings: CopyFcn=set_param(gcbh,'LinkStatus','none');
  evChanges1 : Subsystem
      settings: CopyFcn=set_param(gcbh,'LinkStatus','none');
  notAlways : Subsystem
      settings: CopyFcn=set_param(gcbh,'LinkStatus','none');
  out : Outport  VectorParamsAs1DForOutWhenUnconnected=off
  wires:
  Detect Increase/1 -> evChanges1/3(inputSignal)
  Logical Operator3/1 -> Logical Operator2/2
  Relational Operator2/1 -> Logical Operator3/1
  Relational Operator3/1 -> Logical Operator3/2
  Constant7/1 -> Relational Operator3/2
  Constant6/1 -> Relational Operator2/2
  Abs1/1 -> Unit Delay/1, Relational Operator3/1, Relational Operator1/1
  Logical Operator2/1 -> Detect Increase/1
  Constant2/1 -> Relational Operator1/2
  Logical Operator1/1 -> Logical Operator2/1
  evChanges1/1(evChanges) -> Logical Operator8/3
  Unit Delay/1 -> Relational Operator2/1, Relational Operator4/1
  Constant4/1 -> evChanges1/1(duration)
  Relational Operator1/1 -> Logical Operator1/1
  Constant5/1 -> Relational Operator4/2
  Constant1/1 -> evChanges1/2(sampleTime)
  Relational Operator4/1 -> Logical Operator1/2
  speed/1 -> Abs1/1
  Logical Operator8/1 -> out/1
  Constant8/1 -> notAlways/1(sampleTime)
  PreCond_Eval/1 -> notAlways/3(inputBoolean)
  evChanges/1(evChanges) -> Logical Operator8/2
  notAlways/1(notAlways) -> Logical Operator8/1
  downThreshold/1 -> evChanges/3(inputSignal)
  Constant3/1 -> evChanges/2(sampleTime)
  Constant10/1 -> notAlways/2(timeHorizon)
  Constant11/1 -> evChanges/1(duration)

== system ADI/subsystem1/evChanges ==
  duration : Inport
  sampleTime : Inport  Port=2
  inputSignal : Inport  Port=3
  Constant1 : Constant  Value=0
  Detect Change1 : simulink/Logic and Bit Operations/Detect Change  vinit=0  OutDataTypeStr=boolean
  Relational Operator1 : RelationalOperator  Operator=>  OutDataTypeStr=boolean  RndMeth=Nearest
  Saturation : Saturate  UpperLimit=Inf  LowerLimit=0
  Subtract : Sum  Inputs=-+
  Switch1 : Switch  Criteria=u2 ~= 0
  Unit Delay1 : UnitDelay  SampleTime=-1  HasFrameUpgradeWarning=on
  evChanges : Outport  VectorParamsAs1DForOutWhenUnconnected=off
  wires:
  Detect Change1/1 -> Switch1/2
  duration/1 -> Switch1/1
  Switch1/1 -> Saturation/1
  inputSignal/1 -> Detect Change1/1
  Constant1/1 -> Relational Operator1/2
  Subtract/1 -> Switch1/3
  Saturation/1 -> Relational Operator1/1, Unit Delay1/1
  Unit Delay1/1 -> Subtract/2
  Relational Operator1/1 -> evChanges/1
  sampleTime/1 -> Subtract/1

== system ADI/subsystem2/evChanges ==
  duration : Inport
  sampleTime : Inport  Port=2
  inputSignal : Inport  Port=3
  Constant1 : Constant  Value=0
  Detect Change1 : simulink/Logic and Bit Operations/Detect Change  vinit=0  OutDataTypeStr=boolean
  Relational Operator1 : RelationalOperator  Operator=>  OutDataTypeStr=boolean  RndMeth=Nearest
  Saturation : Saturate  UpperLimit=Inf  LowerLimit=0
  Subtract : Sum  Inputs=-+
  Switch1 : Switch  Criteria=u2 ~= 0
  Unit Delay1 : UnitDelay  SampleTime=-1  HasFrameUpgradeWarning=on
  evChanges : Outport  VectorParamsAs1DForOutWhenUnconnected=off
  wires:
  Detect Change1/1 -> Switch1/2
  duration/1 -> Switch1/1
  Switch1/1 -> Saturation/1
  inputSignal/1 -> Detect Change1/1
  Constant1/1 -> Relational Operator1/2
  Subtract/1 -> Switch1/3
  Saturation/1 -> Relational Operator1/1, Unit Delay1/1
  Unit Delay1/1 -> Subtract/2
  Relational Operator1/1 -> evChanges/1
  sampleTime/1 -> Subtract/1

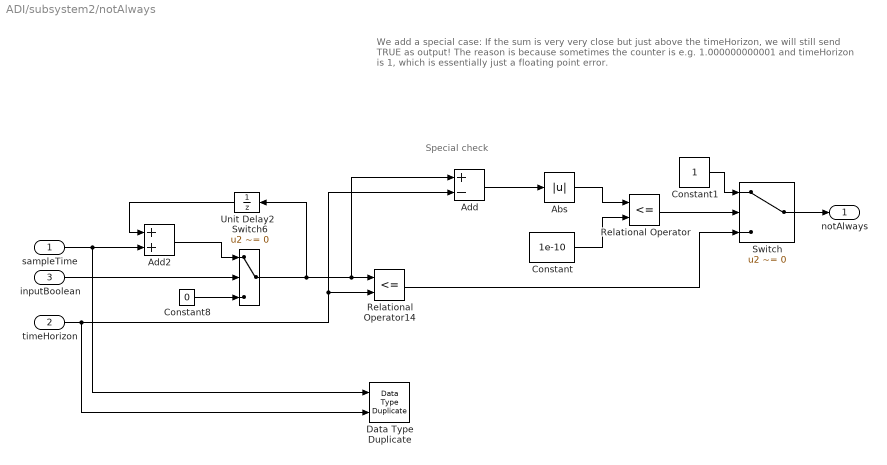
== system ADI/subsystem2/notAlways ==
  note: Special check
  note: We add a special case:
      | If the sum is very very close but just above the timeHorizon, we will still send TRUE as output!
      |
      | The reason is because sometimes the counter is e.g. 1.000000000001 and timeHorizon is 1, which is essentially just a floating point error.
  sampleTime : Inport
  timeHorizon : Inport  Port=2
  inputBoolean : Inport  Port=3
  Abs : Abs
  Add : Sum  Inputs=+-
  Add2 : Sum
  Constant : Constant  Value=1e-10
  Constant1 : Constant  OutDataTypeStr=boolean
  Constant8 : Constant  Value=0  OutDataTypeStr=Inherit: Inherit via back propagation
  Data Type Duplicate : DataTypeDuplicate
  Relational Operator : RelationalOperator  Operator=<=  OutDataTypeStr=boolean  RndMeth=Simplest
  Relational Operator14 : RelationalOperator  Operator=<=  OutDataTypeStr=boolean  RndMeth=Nearest
  Switch : Switch  Criteria=u2 ~= 0
  Switch6 : Switch  Criteria=u2 ~= 0
  Unit Delay2 : UnitDelay  SampleTime=-1  HasFrameUpgradeWarning=on
  notAlways : Outport  VectorParamsAs1DForOutWhenUnconnected=off
  wires:
  Switch6/1 -> Add/1, Relational Operator14/1, Unit Delay2/1
  timeHorizon/1 -> Add/2, Relational Operator14/2, Data Type Duplicate/2
  Relational Operator14/1 -> Switch/3
  Unit Delay2/1 -> Add2/1
  Add2/1 -> Switch6/1
  sampleTime/1 -> Add2/2, Data Type Duplicate/1
  Constant8/1 -> Switch6/3
  inputBoolean/1 -> Switch6/2
  Add/1 -> Abs/1
  Abs/1 -> Relational Operator/1
  Constant/1 -> Relational Operator/2
  Relational Operator/1 -> Switch/2
  Constant1/1 -> Switch/1
  Switch/1 -> notAlways/1

== system ADI/subsystem4/SR_FF ==
  S : Inport  OutDataTypeStr=boolean
  R : Inport  Port=2  OutDataTypeStr=boolean
  LogOp1 : Logic  Tag=struct('inputs','1','comment',struct('text','','placement',1),'logdata',struct('maxnumvals',4096,'plotchannels',[],'loggingmode',3,'channels',1),'operator','NOT','output',struct('class','default','description','','address','','unit','-','name','$S_$B','variable','','type','Bool'),'date',733638.68643228011,'scalingvalid',0)  Operator=NOT  Inputs=1  OutDataTypeStr=boolean
  LogOp2 : Logic  Tag=struct('inputs','2','comment',struct('text','','placement',1),'logdata',struct('maxnumvals',4096,'plotchannels',[],'loggingmode',3,'channels',1),'operator','AND','output',struct('class','default','description','','address','','unit','-','name','$S_$B','variable','','type','Bool'),'date',733638.68643680552,'scalingvalid',0)  Operator=OR  OutDataTypeStr=boolean
  LogOp3 : Logic  Tag=struct('inputs','2','comment',struct('text','','placement',1),'logdata',struct('maxnumvals',4096,'plotchannels',[],'loggingmode',3,'channels',1),'operator','OR','output',struct('class','default','description','','address','','unit','-','name','$S_$B','variable','','type','Bool'),'date',733638.68644151615,'scalingvalid',0)  OutDataTypeStr=boolean
  UnitDelay1 : UnitDelay  Tag=struct('comment',struct('text','','placement',1),'logdata',struct('maxnumvals',4096,'plotchannels',[],'loggingmode',3,'channels',1),'output',struct('width',1,'name','$S_$B','unit','','type','Bool','offset',0,'max',NaN,'min',NaN,'freeze',1,'lsb',1,'arb',0,'class','default','address','','description','','autoscalingmode',1,'lowerheadroom',1,'upperheadroom',1,'headroomunit','bit','checkmin',0,'checkmax',0,'show',0,'variable','','scaling','','keepdatatype',1,'castoutput',0),'state',struct('variable','','description','','name','X_$S_$B','width',1,'address','','max',NaN,'min',NaN,'class','default','type','Bool','scaling','','lsb',1,'offset',0,'arb',0,'freeze',1,'unit','','initial','0'),'dt','-1','date',733638.68644640048,'scalingvalid',0)  SampleTime=-1  HasFrameUpgradeWarning=on
  Q : Outport  OutDataTypeStr=boolean  VectorParamsAs1DForOutWhenUnconnected=off
  wires:
  UnitDelay1/1 -> LogOp2/1  "UnitDelay1_1"
  S/1 -> LogOp2/2
  R/1 -> LogOp1/1
  LogOp2/1 -> LogOp3/1
  LogOp1/1 -> LogOp3/2
  LogOp3/1 -> UnitDelay1/1, Q/1

== system ADI/subsystem4/SR_FF1 ==
  S : Inport  OutDataTypeStr=boolean
  R : Inport  Port=2  OutDataTypeStr=boolean
  LogOp1 : Logic  Tag=struct('inputs','1','comment',struct('text','','placement',1),'logdata',struct('maxnumvals',4096,'plotchannels',[],'loggingmode',3,'channels',1),'operator','NOT','output',struct('class','default','description','','address','','unit','-','name','$S_$B','variable','','type','Bool'),'date',733638.68643228011,'scalingvalid',0)  Operator=NOT  Inputs=1  OutDataTypeStr=boolean
  LogOp2 : Logic  Tag=struct('inputs','2','comment',struct('text','','placement',1),'logdata',struct('maxnumvals',4096,'plotchannels',[],'loggingmode',3,'channels',1),'operator','AND','output',struct('class','default','description','','address','','unit','-','name','$S_$B','variable','','type','Bool'),'date',733638.68643680552,'scalingvalid',0)  Operator=OR  OutDataTypeStr=boolean
  LogOp3 : Logic  Tag=struct('inputs','2','comment',struct('text','','placement',1),'logdata',struct('maxnumvals',4096,'plotchannels',[],'loggingmode',3,'channels',1),'operator','OR','output',struct('class','default','description','','address','','unit','-','name','$S_$B','variable','','type','Bool'),'date',733638.68644151615,'scalingvalid',0)  OutDataTypeStr=boolean
  UnitDelay1 : UnitDelay  Tag=struct('comment',struct('text','','placement',1),'logdata',struct('maxnumvals',4096,'plotchannels',[],'loggingmode',3,'channels',1),'output',struct('width',1,'name','$S_$B','unit','','type','Bool','offset',0,'max',NaN,'min',NaN,'freeze',1,'lsb',1,'arb',0,'class','default','address','','description','','autoscalingmode',1,'lowerheadroom',1,'upperheadroom',1,'headroomunit','bit','checkmin',0,'checkmax',0,'show',0,'variable','','scaling','','keepdatatype',1,'castoutput',0),'state',struct('variable','','description','','name','X_$S_$B','width',1,'address','','max',NaN,'min',NaN,'class','default','type','Bool','scaling','','lsb',1,'offset',0,'arb',0,'freeze',1,'unit','','initial','0'),'dt','-1','date',733638.68644640048,'scalingvalid',0)  SampleTime=-1  HasFrameUpgradeWarning=on
  Q : Outport  OutDataTypeStr=boolean  VectorParamsAs1DForOutWhenUnconnected=off
  wires:
  UnitDelay1/1 -> LogOp2/1  "UnitDelay1_2"
  S/1 -> LogOp2/2
  R/1 -> LogOp1/1
  LogOp2/1 -> LogOp3/1
  LogOp1/1 -> LogOp3/2
  LogOp3/1 -> UnitDelay1/1, Q/1

== system ADI/subsystem4/SR_FF2 ==
  S : Inport  OutDataTypeStr=boolean
  R : Inport  Port=2  OutDataTypeStr=boolean
  LogOp1 : Logic  Tag=struct('inputs','1','comment',struct('text','','placement',1),'logdata',struct('maxnumvals',4096,'plotchannels',[],'loggingmode',3,'channels',1),'operator','NOT','output',struct('class','default','description','','address','','unit','-','name','$S_$B','variable','','type','Bool'),'date',733638.68643228011,'scalingvalid',0)  Operator=NOT  Inputs=1  OutDataTypeStr=boolean
  LogOp2 : Logic  Tag=struct('inputs','2','comment',struct('text','','placement',1),'logdata',struct('maxnumvals',4096,'plotchannels',[],'loggingmode',3,'channels',1),'operator','AND','output',struct('class','default','description','','address','','unit','-','name','$S_$B','variable','','type','Bool'),'date',733638.68643680552,'scalingvalid',0)  Operator=OR  OutDataTypeStr=boolean
  LogOp3 : Logic  Tag=struct('inputs','2','comment',struct('text','','placement',1),'logdata',struct('maxnumvals',4096,'plotchannels',[],'loggingmode',3,'channels',1),'operator','OR','output',struct('class','default','description','','address','','unit','-','name','$S_$B','variable','','type','Bool'),'date',733638.68644151615,'scalingvalid',0)  OutDataTypeStr=boolean
  UnitDelay1 : UnitDelay  Tag=struct('comment',struct('text','','placement',1),'logdata',struct('maxnumvals',4096,'plotchannels',[],'loggingmode',3,'channels',1),'output',struct('width',1,'name','$S_$B','unit','','type','Bool','offset',0,'max',NaN,'min',NaN,'freeze',1,'lsb',1,'arb',0,'class','default','address','','description','','autoscalingmode',1,'lowerheadroom',1,'upperheadroom',1,'headroomunit','bit','checkmin',0,'checkmax',0,'show',0,'variable','','scaling','','keepdatatype',1,'castoutput',0),'state',struct('variable','','description','','name','X_$S_$B','width',1,'address','','max',NaN,'min',NaN,'class','default','type','Bool','scaling','','lsb',1,'offset',0,'arb',0,'freeze',1,'unit','','initial','0'),'dt','-1','date',733638.68644640048,'scalingvalid',0)  SampleTime=-1  HasFrameUpgradeWarning=on
  Q : Outport  OutDataTypeStr=boolean  VectorParamsAs1DForOutWhenUnconnected=off
  wires:
  UnitDelay1/1 -> LogOp2/1
  S/1 -> LogOp2/2
  R/1 -> LogOp1/1
  LogOp2/1 -> LogOp3/1
  LogOp1/1 -> LogOp3/2
  LogOp3/1 -> UnitDelay1/1, Q/1

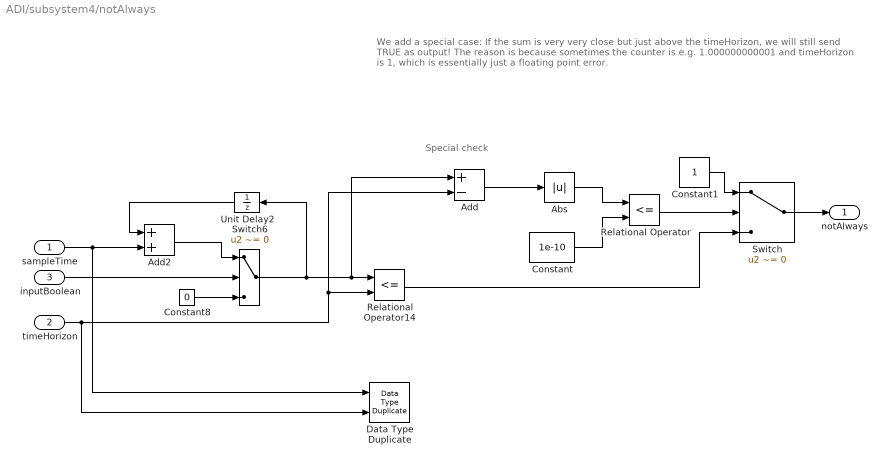
== system ADI/subsystem4/notAlways ==
  note: Special check
  note: We add a special case:
      | If the sum is very very close but just above the timeHorizon, we will still send TRUE as output!
      |
      | The reason is because sometimes the counter is e.g. 1.000000000001 and timeHorizon is 1, which is essentially just a floating point error.
  sampleTime : Inport
  timeHorizon : Inport  Port=2
  inputBoolean : Inport  Port=3
  Abs : Abs
  Add : Sum  Inputs=+-
  Add2 : Sum
  Constant : Constant  Value=1e-10
  Constant1 : Constant  OutDataTypeStr=boolean
  Constant8 : Constant  Value=0  OutDataTypeStr=Inherit: Inherit via back propagation
  Data Type Duplicate : DataTypeDuplicate
  Relational Operator : RelationalOperator  Operator=<=  OutDataTypeStr=boolean  RndMeth=Simplest
  Relational Operator14 : RelationalOperator  Operator=<=  OutDataTypeStr=boolean  RndMeth=Nearest
  Switch : Switch  Criteria=u2 ~= 0
  Switch6 : Switch  Criteria=u2 ~= 0
  Unit Delay2 : UnitDelay  SampleTime=-1  HasFrameUpgradeWarning=on
  notAlways : Outport  VectorParamsAs1DForOutWhenUnconnected=off
  wires:
  Switch6/1 -> Add/1, Relational Operator14/1, Unit Delay2/1
  timeHorizon/1 -> Add/2, Relational Operator14/2, Data Type Duplicate/2
  Relational Operator14/1 -> Switch/3
  Unit Delay2/1 -> Add2/1
  Add2/1 -> Switch6/1
  sampleTime/1 -> Add2/2, Data Type Duplicate/1
  Constant8/1 -> Switch6/3
  inputBoolean/1 -> Switch6/2
  Add/1 -> Abs/1
  Abs/1 -> Relational Operator/1
  Constant/1 -> Relational Operator/2
  Relational Operator/1 -> Switch/2
  Constant1/1 -> Switch/1
  Switch/1 -> notAlways/1

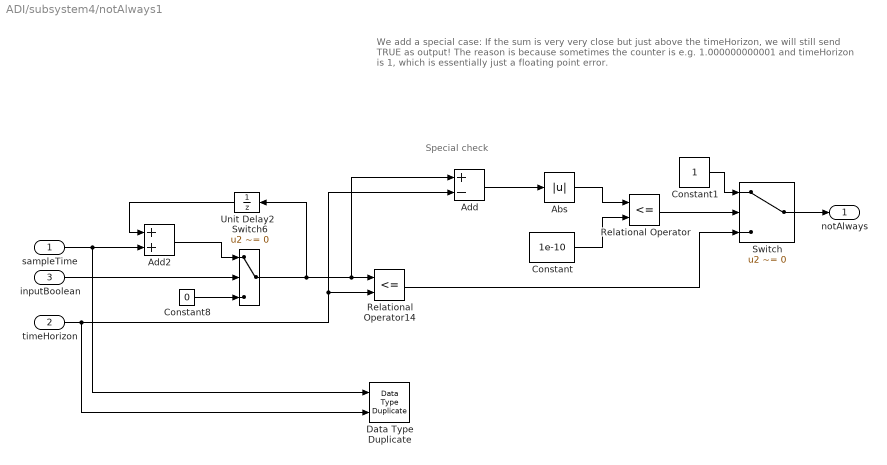
== system ADI/subsystem4/notAlways1 ==
  note: Special check
  note: We add a special case:
      | If the sum is very very close but just above the timeHorizon, we will still send TRUE as output!
      |
      | The reason is because sometimes the counter is e.g. 1.000000000001 and timeHorizon is 1, which is essentially just a floating point error.
  sampleTime : Inport
  timeHorizon : Inport  Port=2
  inputBoolean : Inport  Port=3
  Abs : Abs
  Add : Sum  Inputs=+-
  Add2 : Sum
  Constant : Constant  Value=1e-10
  Constant1 : Constant  OutDataTypeStr=boolean
  Constant8 : Constant  Value=0  OutDataTypeStr=Inherit: Inherit via back propagation
  Data Type Duplicate : DataTypeDuplicate
  Relational Operator : RelationalOperator  Operator=<=  OutDataTypeStr=boolean  RndMeth=Simplest
  Relational Operator14 : RelationalOperator  Operator=<=  OutDataTypeStr=boolean  RndMeth=Nearest
  Switch : Switch  Criteria=u2 ~= 0
  Switch6 : Switch  Criteria=u2 ~= 0
  Unit Delay2 : UnitDelay  SampleTime=-1  HasFrameUpgradeWarning=on
  notAlways : Outport  VectorParamsAs1DForOutWhenUnconnected=off
  wires:
  Switch6/1 -> Add/1, Relational Operator14/1, Unit Delay2/1
  timeHorizon/1 -> Add/2, Relational Operator14/2, Data Type Duplicate/2
  Relational Operator14/1 -> Switch/3
  Unit Delay2/1 -> Add2/1
  Add2/1 -> Switch6/1
  sampleTime/1 -> Add2/2, Data Type Duplicate/1
  Constant8/1 -> Switch6/3
  inputBoolean/1 -> Switch6/2
  Add/1 -> Abs/1
  Abs/1 -> Relational Operator/1
  Constant/1 -> Relational Operator/2
  Relational Operator/1 -> Switch/2
  Constant1/1 -> Switch/1
  Switch/1 -> notAlways/1

== system ADI/subsystem5/evChanges ==
  duration : Inport
  sampleTime : Inport  Port=2
  inputSignal : Inport  Port=3
  Constant1 : Constant  Value=0
  Detect Change1 : simulink/Logic and Bit Operations/Detect Change  vinit=0  OutDataTypeStr=boolean
  Relational Operator1 : RelationalOperator  Operator=>  OutDataTypeStr=boolean  RndMeth=Nearest
  Saturation : Saturate  UpperLimit=Inf  LowerLimit=0
  Subtract : Sum  Inputs=-+
  Switch1 : Switch  Criteria=u2 ~= 0
  Unit Delay1 : UnitDelay  SampleTime=-1  HasFrameUpgradeWarning=on
  evChanges : Outport  VectorParamsAs1DForOutWhenUnconnected=off
  wires:
  Detect Change1/1 -> Switch1/2
  duration/1 -> Switch1/1
  Switch1/1 -> Saturation/1
  inputSignal/1 -> Detect Change1/1
  Constant1/1 -> Relational Operator1/2
  Subtract/1 -> Switch1/3
  Saturation/1 -> Relational Operator1/1, Unit Delay1/1
  Unit Delay1/1 -> Subtract/2
  Relational Operator1/1 -> evChanges/1
  sampleTime/1 -> Subtract/1

== system ADI/subsystem5/evChanges1 ==
  duration : Inport
  sampleTime : Inport  Port=2
  inputSignal : Inport  Port=3
  Constant1 : Constant  Value=0
  Detect Change1 : simulink/Logic and Bit Operations/Detect Change  vinit=0  OutDataTypeStr=boolean
  Relational Operator1 : RelationalOperator  Operator=>  OutDataTypeStr=boolean  RndMeth=Nearest
  Saturation : Saturate  UpperLimit=Inf  LowerLimit=0
  Subtract : Sum  Inputs=-+
  Switch1 : Switch  Criteria=u2 ~= 0
  Unit Delay1 : UnitDelay  SampleTime=-1  HasFrameUpgradeWarning=on
  evChanges : Outport  VectorParamsAs1DForOutWhenUnconnected=off
  wires:
  Detect Change1/1 -> Switch1/2
  duration/1 -> Switch1/1
  Switch1/1 -> Saturation/1
  inputSignal/1 -> Detect Change1/1
  Constant1/1 -> Relational Operator1/2
  Subtract/1 -> Switch1/3
  Saturation/1 -> Relational Operator1/1, Unit Delay1/1
  Unit Delay1/1 -> Subtract/2
  Relational Operator1/1 -> evChanges/1
  sampleTime/1 -> Subtract/1

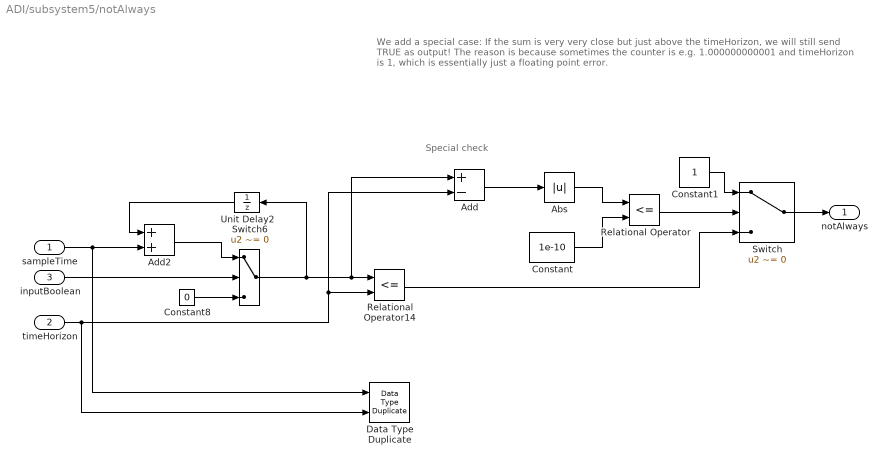
== system ADI/subsystem5/notAlways ==
  note: Special check
  note: We add a special case:
      | If the sum is very very close but just above the timeHorizon, we will still send TRUE as output!
      |
      | The reason is because sometimes the counter is e.g. 1.000000000001 and timeHorizon is 1, which is essentially just a floating point error.
  sampleTime : Inport
  timeHorizon : Inport  Port=2
  inputBoolean : Inport  Port=3
  Abs : Abs
  Add : Sum  Inputs=+-
  Add2 : Sum
  Constant : Constant  Value=1e-10
  Constant1 : Constant  OutDataTypeStr=boolean
  Constant8 : Constant  Value=0  OutDataTypeStr=Inherit: Inherit via back propagation
  Data Type Duplicate : DataTypeDuplicate
  Relational Operator : RelationalOperator  Operator=<=  OutDataTypeStr=boolean  RndMeth=Simplest
  Relational Operator14 : RelationalOperator  Operator=<=  OutDataTypeStr=boolean  RndMeth=Nearest
  Switch : Switch  Criteria=u2 ~= 0
  Switch6 : Switch  Criteria=u2 ~= 0
  Unit Delay2 : UnitDelay  SampleTime=-1  HasFrameUpgradeWarning=on
  notAlways : Outport  VectorParamsAs1DForOutWhenUnconnected=off
  wires:
  Switch6/1 -> Add/1, Relational Operator14/1, Unit Delay2/1
  timeHorizon/1 -> Add/2, Relational Operator14/2, Data Type Duplicate/2
  Relational Operator14/1 -> Switch/3
  Unit Delay2/1 -> Add2/1
  Add2/1 -> Switch6/1
  sampleTime/1 -> Add2/2, Data Type Duplicate/1
  Constant8/1 -> Switch6/3
  inputBoolean/1 -> Switch6/2
  Add/1 -> Abs/1
  Abs/1 -> Relational Operator/1
  Constant/1 -> Relational Operator/2
  Relational Operator/1 -> Switch/2
  Constant1/1 -> Switch/1
  Switch/1 -> notAlways/1
